simulink model "main_sim"  (R2015a)
settings: Solver=ode3  StartTime=0.0  StopTime=0.04  FixedStep=0.00001  RelTol=1e-4
InitFcn:
  | params;
  | init_non_lin;
  | init_lin;
StopFcn:
  | compar_lin_nonlin
  | %visualisation_sim
values from neighbouring files (symbols this model uses):
  A1 = i_w+m_w*(R^2)+m_r*(R^2)    [init_non_lin.m]
  A2 = i_r +m_r*L^2    [init_non_lin.m]
  Ac = [ 0       0          1     0 ... (first row only)    [init_lin.m]
  Ad = sys_d.A    [init_lin.m]
  B1 = m_r*R*L    [init_non_lin.m]
  B2 = m_r*R*L    [init_non_lin.m]
  Bc = [0; 0; -((E^-1)*H)]    [init_lin.m]
  Bd = sys_d.B    [init_lin.m]
  C1 = m_r*R*L    [init_non_lin.m]
  C2 = m_r*g*L    [init_non_lin.m]
  Cc = [0 0 R 0 ... (first row only)    [init_lin.m]
  Cd = sys_d.C    [init_lin.m]
  dt = 0.005    [params.m]
  x_0 = [0.01;0.01;0;0]    [init_lin.m]
libraries: simulink x5
settings Model: Creator=Monika  LastModifiedBy=Michał

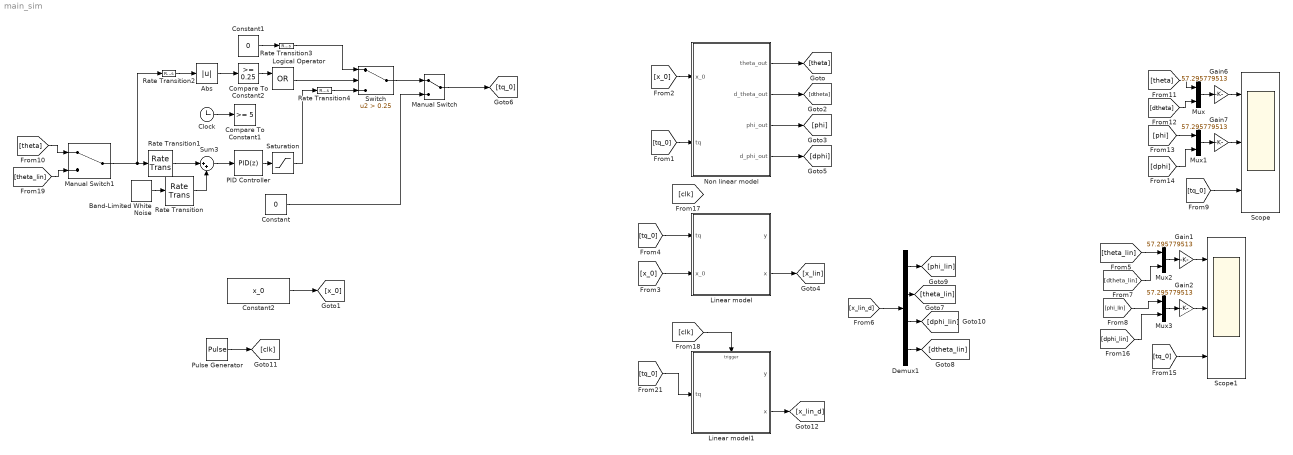
== system main_sim ==
  Abs : Abs
  Band-Limited White Noise : simulink/Sources/Band-Limited White Noise  Cov=1e-9  Ts=0.001  seed=[23341]
  Clock : Clock
  Compare To Constant1 : simulink/Logic and Bit Operations/Compare To Constant  relop=>=  const=5  OutDataTypeStr=boolean
  Compare To Constant2 : simulink/Logic and Bit Operations/Compare To Constant  relop=>=  const=0.25  OutDataTypeStr=boolean
  Constant : Constant  Value=0
  Constant1 : Constant  Value=0
  Constant2 : Constant  Value=x_0
  Demux1 : Demux
  Gain{1..2,6..7} (4 alike) : Gain  Gain=57.295779513
  Linear model : Subsystem
  Linear model1 : Subsystem
      settings: MinAlgLoopOccurrences=on
  Logical Operator : Logic  Operator=OR  AllPortsSameDT=off  OutDataTypeStr=boolean
  Manual Switch : ManualSwitch
  Manual Switch1 : ManualSwitch
  Mux{,1..3} (4 alike) : Mux  Inputs=2
  Non linear model : Subsystem
  PID Controller : simulink/Continuous/PID Controller  Controller=PID  TimeDomain=Discrete-time  SampleTime=0.001  IntegratorMethod=Trapezoidal  FilterMethod=Forward Euler  Form=Parallel  UseFilter=off  ControllerParametersSource=internal  P=60  I=6  D=5  N=460.807410242904  InitialConditionSource=internal  InitialConditionForIntegrator=0  InitialConditionForFilter=0  ExternalReset=none  LimitOutput=off  UpperSaturationLimit=inf  LowerSaturationLimit=-inf  LinearizeAsGain=on  AntiWindupMode=none  Kb=1  TrackingMode=off  Kt=1  PParamMin=[]  PParamMax=[]  IParamMin=[]  IParamMax=[]  DParamMin=[]  DParamMax=[]  NParamMin=[]  NParamMax=[]  KbParamMin=[]  KbParamMax=[]  KtParamMin=[]  KtParamMax=[]  POutMin=[]  POutMax=[]  IOutMin=[]  IOutMax=[]  DOutMin=[]  DOutMax=[]  NOutMin=[]  NOutMax=[]  KbOutMin=[]  KbOutMax=[]  KtOutMin=[]  KtOutMax=[]  IntegratorOutMin=[]  IntegratorOutMax=[]  FilterOutMin=[]  FilterOutMax=[]  SumOutMin=[]  SumOutMax=[]  SumI1OutMin=[]  SumI1OutMax=[]  SumI2OutMin=[]  SumI2OutMax=[]  SumI3OutMin=[]  SumI3OutMax=[]  SumDOutMin=[]  SumDOutMax=[]  SaturationOutMin=[]  SaturationOutMax=[]  IntegratorContinuousStateAttributes=''  IntegratorStateMustResolveToSignalObject=off  IntegratorRTWStateStorageClass=Auto  FilterContinuousStateAttributes=''  FilterStateMustResolveToSignalObject=off  FilterRTWStateStorageClass=Auto  DifferentiatorICPrevScaledInput=0  DifferentiatorOutMin=[]  DifferentiatorOutMax=[]
  Pulse Generator : DiscretePulseGenerator  PulseType=Time based  Period=dt  PulseWidth=50
  Rate Transition : RateTransition
  Rate Transition1 : RateTransition  OutPortSampleTime=0.001
  Rate Transition2 : RateTransition  OutPortSampleTime=0.00001
  Rate Transition3 : RateTransition  Integrity=off  Deterministic=off  OutPortSampleTimeMultiple=0.001  OutPortSampleTime=0.00001
  Rate Transition4 : RateTransition  Integrity=off  Deterministic=off  OutPortSampleTimeMultiple=0.001  OutPortSampleTime=0.00001
  Saturation : Saturate  UpperLimit=0.3  LowerLimit=-0.3
  Scope : Scope  NumInputPorts=3
      settings: TimeRange=60  YMin=-2~-4~-1  YMax=8~4~1  SaveName=sim_out_nonlin
  Scope1 : Scope  NumInputPorts=3
      settings: TimeRange=10  YMin=-6016.06~2250~-1  YMax=-5443.1~5750~1  SaveName=sim_out_lin
  Sum3 : Sum  Inputs=|++
  Switch : Switch  Criteria=u2 > Threshold  Threshold=0.25
  wires:
  Mux1/1 -> Gain7/1
  [tq_0] -> Scope/3
  Constant/1 -> Manual Switch/2
  PID Controller/1 -> Saturation/1
  Manual Switch/1 -> [tq_0]
  Sum3/1 -> PID Controller/1
  Band-Limited White Noise/1 -> Rate Transition/1
  Switch/1 -> Manual Switch/1
  Saturation/1 -> Rate Transition4/1
  Abs/1 -> Compare To Constant2/1
  Constant1/1 -> Rate Transition3/1
  [theta] -> Mux/1
  [dtheta] -> Mux/2
  [phi] -> Mux1/1
  [dphi] -> Mux1/2
  Clock/1 -> Compare To Constant1/1
  Logical Operator/1 -> Switch/2
  Compare To Constant2/1 -> Logical Operator/1
  Mux/1 -> Gain6/1
  Rate Transition/1 -> Sum3/2
  Gain6/1 -> Scope/1
  Gain7/1 -> Scope/2
  [tq_0] -> Non linear model/2(tq)
  Constant2/1 -> [x_0]
  [x_0] -> Non linear model/1(x_0)
  Non linear model/1(theta_out) -> [theta]
  Non linear model/2(d_theta_out) -> [dtheta]
  Non linear model/3(phi_out) -> [phi]
  Non linear model/4(d_phi_out) -> [dphi]
  [x_0] -> Linear model/2(x_0)
  [tq_0] -> Linear model/1(tq)
  Linear model/2(x) -> [x_lin]
  Mux3/1 -> Gain2/1
  [tq_0] -> Scope1/3
  Mux2/1 -> Gain1/1
  Gain1/1 -> Scope1/1
  Gain2/1 -> Scope1/2
  Rate Transition2/1 -> Abs/1
  Rate Transition3/1 -> Switch/1
  Rate Transition4/1 -> Switch/3
  Demux1/2 -> [theta_lin]
  Demux1/4 -> [dtheta_lin]
  Demux1/1 -> [phi_lin]
  Demux1/3 -> [dphi_lin]
  [theta_lin] -> Mux2/1
  [dtheta_lin] -> Mux2/2
  [phi_lin] -> Mux3/1
  [dphi_lin] -> Mux3/2
  Pulse Generator/1 -> [clk]
  [theta] -> Manual Switch1/1
  [theta_lin] -> Manual Switch1/2
  Manual Switch1/1 -> Rate Transition2/1, Rate Transition1/1
  Rate Transition1/1 -> Sum3/1
  [tq_0] -> Linear model1/1(tq)
  Linear model1/2(x) -> [x_lin_d]
  [clk] -> Linear model1/Trigger
  [x_lin_d] -> Demux1/1

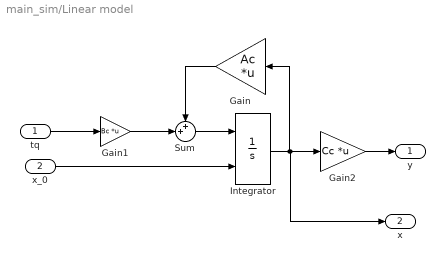
== system main_sim/Linear model ==
  tq : Inport
  x_0 : Inport  Port=2
  Gain : Gain  Gain=Ac  Multiplication=Matrix(K*u) (u vector)
  Gain1 : Gain  Gain=Bc  Multiplication=Matrix(K*u) (u vector)
  Gain2 : Gain  Gain=Cc  Multiplication=Matrix(K*u) (u vector)
  Integrator : Integrator  InitialConditionSource=external  UpperSaturationLimit=100  LowerSaturationLimit=-100
  Sum : Sum  Inputs=++|
  y : Outport
  x : Outport  Port=2
  wires:
  Gain2/1 -> y/1
  x_0/1 -> Integrator/2
  Integrator/1 -> Gain/1, x/1, Gain2/1
  Gain/1 -> Sum/1
  Gain1/1 -> Sum/2
  Sum/1 -> Integrator/1
  tq/1 -> Gain1/1

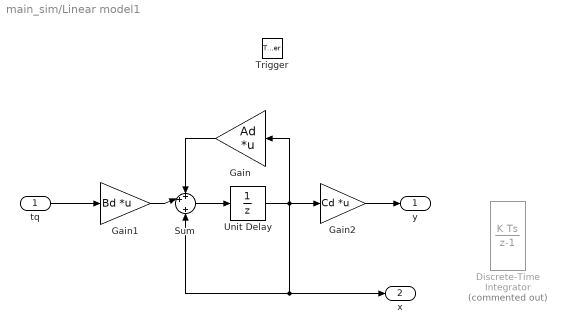
== system main_sim/Linear model1 ==
  tq : Inport
  Trigger : TriggerPort  PortDimensions=1
  Discrete-Time Integrator : DiscreteIntegrator  Commented=on  InitialConditionSource=external  SampleTime=-1
  Gain : Gain  Gain=Ad  Multiplication=Matrix(K*u) (u vector)
  Gain1 : Gain  Gain=Bd  Multiplication=Matrix(K*u) (u vector)
  Gain2 : Gain  Gain=Cd  Multiplication=Matrix(K*u) (u vector)
  Sum : Sum  Inputs=++|+
  Unit Delay : UnitDelay  InitialCondition=x_0  SampleTime=-1
  y : Outport
  x : Outport  Port=2
  wires:
  Gain2/1 -> y/1
  Unit Delay/1 -> Gain2/1, x/1, Sum/3, Gain/1
  Gain/1 -> Sum/1
  Gain1/1 -> Sum/2
  Sum/1 -> Unit Delay/1
  tq/1 -> Gain1/1

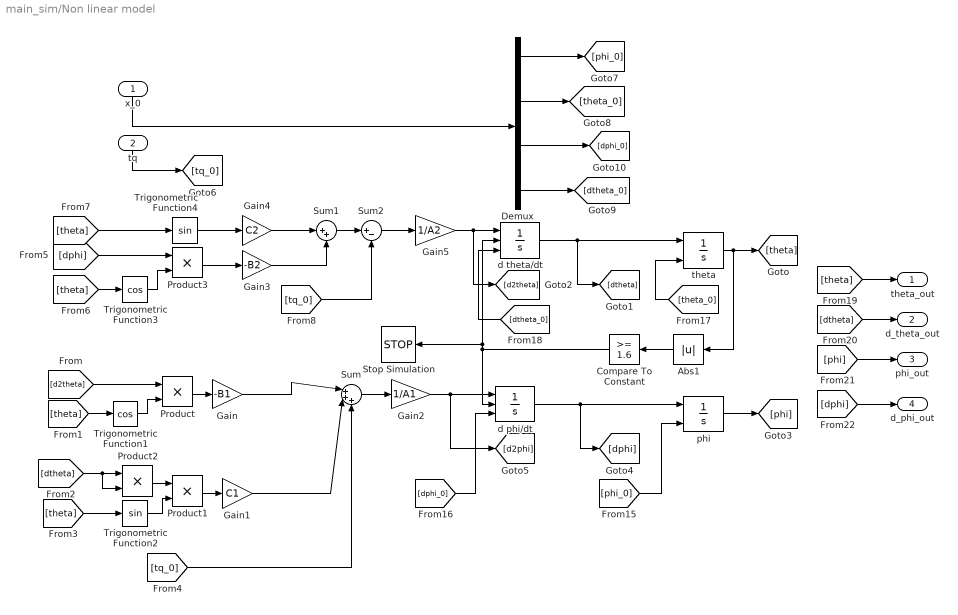
== system main_sim/Non linear model ==
  x_0 : Inport
  tq : Inport  Port=2
  Abs1 : Abs
  Compare To Constant : simulink/Logic and Bit Operations/Compare To Constant  relop=>=  const=1.6  OutDataTypeStr=boolean
  Demux : Demux
  Gain : Gain  Gain=-B1
  Gain1 : Gain  Gain=C1
  Gain2 : Gain  Gain=1/A1
  Gain3 : Gain  Gain=-B2
  Gain4 : Gain  Gain=C2
  Gain5 : Gain  Gain=1/A2
  Product{,1..3} (4 alike) : Product
  Stop Simulation : Stop
  Sum : Sum  Inputs=|+++
  Sum1 : Sum  Inputs=|++
  Sum2 : Sum  Inputs=|+-
  Trigonometric Function1 : Trigonometry  Operator=cos
  Trigonometric Function2 : Trigonometry
  Trigonometric Function3 : Trigonometry  Operator=cos
  Trigonometric Function4 : Trigonometry
  d phi/dt : Integrator  ExternalReset=level  InitialConditionSource=external  UpperSaturationLimit=18  LowerSaturationLimit=-18
  d theta/dt : Integrator  ExternalReset=level  InitialConditionSource=external
  phi : Integrator  InitialConditionSource=external
  theta : Integrator  InitialConditionSource=external  InitialCondition=0.1745329  LimitOutput=on  UpperSaturationLimit=1.6  LowerSaturationLimit=-1.6
  theta_out : Outport
  d_theta_out : Outport  Port=2
  phi_out : Outport  Port=3
  d_phi_out : Outport  Port=4
  wires:
  phi/1 -> [phi]
  d theta/dt/1 -> theta/1, [dtheta]
  [theta] -> Trigonometric Function1/1
  d phi/dt/1 -> phi/1, [dphi]
  Product/1 -> Gain/1
  Trigonometric Function1/1 -> Product/2
  theta/1 -> [theta], Abs1/1
  Demux/3 -> [dphi_0]
  Demux/2 -> [theta_0]
  x_0/1 -> Demux/1
  Demux/4 -> [dtheta_0]
  [theta_0] -> theta/2
  [dphi_0] -> d phi/dt/3
  [dtheta] -> d_theta_out/1
  [phi] -> phi_out/1
  [dphi] -> d_phi_out/1
  [theta] -> theta_out/1
  [dtheta_0] -> d theta/dt/3
  Demux/1 -> [phi_0]
  [phi_0] -> phi/2
  Abs1/1 -> Compare To Constant/1
  Gain5/1 -> [d2theta], d theta/dt/1
  Compare To Constant/1 -> Stop Simulation/1, d theta/dt/2, d phi/dt/2
  Gain1/1 -> Sum/2
  Gain4/1 -> Sum1/1
  Product1/1 -> Gain1/1
  Trigonometric Function2/1 -> Product1/2
  [tq_0] -> Sum/3
  Product3/1 -> Gain3/1
  Sum1/1 -> Sum2/1
  [tq_0] -> Sum2/2
  Gain/1 -> Sum/1
  Sum/1 -> Gain2/1
  Gain3/1 -> Sum1/2
  [dtheta] -> Product2/2, Product2/1
  Gain2/1 -> [d2phi], d phi/dt/1
  [theta] -> Trigonometric Function3/1
  [theta] -> Trigonometric Function4/1
  Trigonometric Function4/1 -> Gain4/1
  Product2/1 -> Product1/1
  [dphi] -> Product3/1
  [d2theta] -> Product/1
  [theta] -> Trigonometric Function2/1
  Trigonometric Function3/1 -> Product3/2
  Sum2/1 -> Gain5/1
  tq/1 -> [tq_0]
